simulink model "UPQC_original"  (R2020a)
settings: Solver=ode45  StartTime=0.0  StopTime=0.3  FixedStep=Ts  RelTol=1e-3  EnableMultiTasking=on
undefined symbols (not defined in the file or in its folder): DiscIntNeverNeededParam, Hydride, level, Metal, Nickel, sigbuilder_block
libraries: powerlib x73, powerlib_extras x9, simulink x7, powerlib_meascontrol x2, electricdrivelib x1, re_lib x1
(part 1 of 3)
settings Model: Creator=Dhamodharan  LastModifiedBy=User
settings DataIOCC: LimitDataPoints=on  SaveFormat=Array  ReturnWorkspaceOutputs=off
settings OptimizationCC: ExpressionDepthLimit=2147483647  InitFltsAndDblsToZero=on  LifeSpan=inf
settings DebuggingCC: SaveWithParameterizedLinksMsg=none  UnderspecifiedInitializationDetection=Classic  MergeDetectMultiDrivingBlocksExec=none  SignalResolutionControl=TryResolveAllWithWarning  SolverPrmCheckMsg=warning  MultiTaskDSMMsg=warning  MultiTaskCondExecSysMsg=none  FcnCallInpInsideContextMsg=warning  StateNameClashWarn=warning  SFUnexpectedBacktrackingDiag=warning  SFNoUnconditionalDefaultTransitionDiag=warning  SFExecutionAtInitializationDiag=none  ArithmeticOperatorsInVariantConditions=warning
settings HardwareCC: ProdBitPerPointer=32  ProdBitPerSizeT=32  ProdBitPerPtrDiffT=32  ProdLargestAtomicFloat=None  ProdIntDivRoundTo=Undefined  ProdEndianess=Unspecified  ProdWordSize=32  ProdHWDeviceType=32-bit Generic
settings ModelReferenceCC: PropagateSignalLabelsOutOfModel=off
settings SFSimCC: SimUseLocalCustomCode=off  CustomCodeUndefinedFunction=UseInterfaceOnly
settings RTWCC: RTWUseLocalCustomCode=off
settings CodeAppCC: StateflowObjectComments=on
settings GRTTargetCC: TargetFcnLib=ansi_tfl_tmw.mat  TargetLangStandard=C89/C90 (ANSI)  CombineOutputUpdateFcns=off  GRTInterface=on
settings ConfigComp: CovMetricSettings=dw  CovHtmlReporting=on  CovSaveCumulativeToWorkspaceVar=on  CovSaveSingleToWorkspaceVar=on  CovExternalEMLEnable=off
settings SimscapeCC: SimscapeNormalizeSystem=off

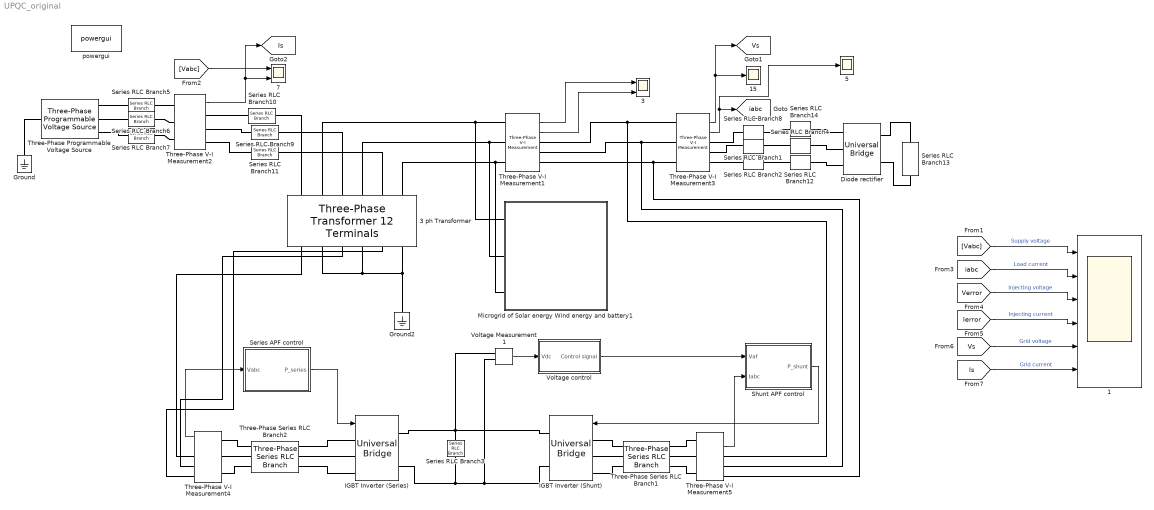
== system UPQC_original ==
  " IGBT Inverter (Series)" : powerlib/Power Electronics/Universal Bridge  Arms=3  SnubberResistance=5000  SnubberCapacitance=1e-6  Device=MOSFET / Diodes  Ron=1e-3  Lon=0  ForwardVoltages="[  0.1  0.1  ]"  ForwardVoltage=.8  GTOparameters=[ 1e-6 ,1e-6 ]  IGBTparameters=[ 1e-6 , 2e-6 ]  Measurements=Device currents  Measurements_2=None  converterType=Rectifier
  1 : Scope  NumInputPorts=6
  15 : Scope
  3 : Scope  NumInputPorts=2
  3 ph Transformer : powerlib/Elements/Three-Phase Transformer 12 Terminals  RatedPower=[ 10e6 50 ]  Winding1="[ 100 0.002  0.00005 ]"  Winding2=[ 100 0.002 0.00005]  RmXm=[ 200 200 ]
      settings: SourceProductBaseCode=PS
  5 : Scope
  7 : Scope  NumInputPorts=2
  Diode rectifier : powerlib/Power Electronics/Universal Bridge  Arms=3  SnubberResistance=1e5  SnubberCapacitance=inf  Device=Diodes  Ron=1e-3  Lon=0  ForwardVoltages="[  0  0  ]"  ForwardVoltage=0  GTOparameters=[ 10e-6 , 20e-6 ]  IGBTparameters=[ 1e-6 , 2e-6 ]  Measurements=None  Measurements_2=None  converterType=Rectifier
  Ground : powerlib/Elements/Ground  LConnTagsString=a
  Ground2 : powerlib/Elements/Ground  LConnTagsString=a
  IGBT Inverter (Shunt) : powerlib/Power Electronics/Universal Bridge  Arms=3  SnubberResistance=5000  SnubberCapacitance=1e-6  Device=MOSFET / Diodes  Ron=1e-3  Lon=0  ForwardVoltages="[  0.1  0.1  ]"  ForwardVoltage=.8  GTOparameters=[ 1e-6 ,1e-6 ]  IGBTparameters=[ 1e-6 , 2e-6 ]  Measurements=Device currents  Measurements_2=None  converterType=Rectifier
  Microgrid of Solar energy Wind energy and battery1 : Subsystem
  Series APF control : Subsystem
  Series RLC Branch{1..2,4,8,12,14} (6 alike) : powerlib/Elements/Series RLC Branch  LConnTagsString=__new0  RConnTagsString=__new0  BranchType=L  Resistance=1.0  Inductance=2e-3  SetiL0=off  InitialCurrent=0  Capacitance=1.0  Setx0=off  InitialVoltage=0  Measurements=None
  Series RLC Branch10 : powerlib/Elements/Series RLC Branch  LConnTagsString=__new0  RConnTagsString=__new0  BranchType=RL  Resistance=0.001  Inductance=1e-5  SetiL0=off  InitialCurrent=0  Capacitance=1.0  Setx0=off  InitialVoltage=0  Measurements=None
  Series RLC Branch11 : powerlib/Elements/Series RLC Branch  LConnTagsString=__new0  RConnTagsString=__new0  BranchType=RL  Resistance=0.001  Inductance=1e-5  SetiL0=off  InitialCurrent=0  Capacitance=1.0  Setx0=off  InitialVoltage=0  Measurements=None
  Series RLC Branch13 : powerlib/Elements/Series RLC Branch  LConnTagsString=__new0  RConnTagsString=__new0  BranchType=R  Resistance=40  Inductance=1e-4  SetiL0=off  InitialCurrent=0  Capacitance=1.0  Setx0=off  InitialVoltage=0  Measurements=None
  Series RLC Branch3 : powerlib/Elements/Series RLC Branch  LConnTagsString=__new0  RConnTagsString=__new0  BranchType=C  Resistance=1.0  Inductance=1.0  SetiL0=off  InitialCurrent=0  Capacitance=5  Setx0=on  InitialVoltage=800  Measurements=None
  Series RLC Branch5 : powerlib/Elements/Series RLC Branch  LConnTagsString=__new0  RConnTagsString=__new0  BranchType=R  Resistance=0.001  Inductance=1.0e-4  SetiL0=off  InitialCurrent=0  Capacitance=1.0  Setx0=off  InitialVoltage=0  Measurements=None
  Series RLC Branch6 : powerlib/Elements/Series RLC Branch  LConnTagsString=__new0  RConnTagsString=__new0  BranchType=R  Resistance=0.001  Inductance=1.0e-4  SetiL0=off  InitialCurrent=0  Capacitance=1.0  Setx0=off  InitialVoltage=0  Measurements=None
  Series RLC Branch7 : powerlib/Elements/Series RLC Branch  LConnTagsString=__new0  RConnTagsString=__new0  BranchType=R  Resistance=0.001  Inductance=1.0e-4  SetiL0=off  InitialCurrent=0  Capacitance=1.0  Setx0=off  InitialVoltage=0  Measurements=None
  Series RLC Branch9 : powerlib/Elements/Series RLC Branch  LConnTagsString=__new0  RConnTagsString=__new0  BranchType=RL  Resistance=0.001  Inductance=1e-5  SetiL0=off  InitialCurrent=0  Capacitance=1.0  Setx0=off  InitialVoltage=0  Measurements=None
  Shunt APF control : Subsystem
  Three-Phase Programmable Voltage Source : powerlib/Electrical Sources/Three-Phase Programmable Voltage Source  PositiveSequence="[230*sqrt(3)/sqrt(2)  0 50]"  VariationEntity=Amplitude  VariationType=Table of time-amplitude pairs  VariationTypeAlt=Step  VariationStep=0.5  VariationRate=10  VariationMagnitude=0.3  VariationFrequency=2  VariationTiming=[1 2]  VariationPhaseA=off  Amplitudes=[1 0.8 1.2 1]  TimeValues=[0 0.1 0.15 0.2]  HarmonicGeneration=on  HarmonicA=[5 0.2 -25 2]  HarmonicB=[7 0.2 35 1]  Timing="[0.25  0.4]"  BusType=swing  Pref=0  Qref=0  Qmin=-inf  Qmax=inf
  Three-Phase Series RLC Branch1 : powerlib/Elements/Three-Phase Series RLC Branch  LConnTagsString=A|B|C  RConnTagsString=A|B|C  BranchType=L  Resistance=0.  Inductance=3e-3  Capacitance=1e-6  Measurements=None
  Three-Phase Series RLC Branch2 : powerlib/Elements/Three-Phase Series RLC Branch  LConnTagsString=A|B|C  RConnTagsString=A|B|C  BranchType=L  Resistance=0.  Inductance=1e-3  Capacitance=1e-6  Measurements=None
  Three-Phase V-I Measurement1 : powerlib/Measurements/Three-Phase V-I Measurement  VoltageMeasurement=phase-to-ground  SetLabelV=off  LabelV=Vabc  Vpu=off  VpuLL=off  CurrentMeasurement=yes  SetLabelI=off  LabelI=Iabc  Ipu=off  Pbase=100e6  Vbase=500e3  OutputType=Complex  PhasorSimulation=off  PSBequivalent=0
  Three-Phase V-I Measurement2 : powerlib/Measurements/Three-Phase V-I Measurement  VoltageMeasurement=phase-to-ground  SetLabelV=on  LabelV=Vabc  Vpu=off  VpuLL=off  CurrentMeasurement=yes  SetLabelI=off  LabelI=Iabc  Ipu=off  Pbase=100e6  Vbase=500e3  OutputType=Complex  PhasorSimulation=off  PSBequivalent=0
  Three-Phase V-I Measurement3 : powerlib/Measurements/Three-Phase V-I Measurement  VoltageMeasurement=phase-to-ground  SetLabelV=off  LabelV=Vabc  Vpu=off  VpuLL=off  CurrentMeasurement=yes  SetLabelI=off  LabelI=Iabc  Ipu=off  Pbase=100e6  Vbase=500e3  OutputType=Complex  PhasorSimulation=off  PSBequivalent=0
  Three-Phase V-I Measurement4 : powerlib/Measurements/Three-Phase V-I Measurement  VoltageMeasurement=phase-to-ground  SetLabelV=off  LabelV=Vabc  Vpu=off  VpuLL=off  CurrentMeasurement=yes  SetLabelI=off  LabelI=Iabc  Ipu=off  Pbase=100e6  Vbase=500e3  OutputType=Complex  PhasorSimulation=off  PSBequivalent=0
  Three-Phase V-I Measurement5 : powerlib/Measurements/Three-Phase V-I Measurement  VoltageMeasurement=phase-to-phase  SetLabelV=off  LabelV=Vabc  Vpu=off  VpuLL=off  CurrentMeasurement=yes  SetLabelI=off  LabelI=Iabc  Ipu=off  Pbase=100e6  Vbase=500e3  OutputType=Complex  PhasorSimulation=off  PSBequivalent=0
  Voltage Measurement1 : powerlib/Measurements/Voltage Measurement  PhasorSimulation=off  OutputType=Complex  PSBequivalent=0
  Voltage control : Subsystem
  powergui : powerlib/powergui  SimulationMode=Discrete  SampleTime=8e-6  frequency=60  Iterations=50  frequencyindice=0  Pbase=100e6  ErrMax=1e-4  UnitsV=kV  UnitsW=MW  buscounter=0  FunctionMessages=off  echomessages=off  EnableUseOfTLC=off  CurrentSourceSwitches=off  DisableSnubberDevices=off  DisableRonSwitches=off  DisableVfSwitches=off  DisplayEquations=off  AutomaticDiscreteSolvers=off  SolverType=Tustin  Interpol=off  ExternalGateDelay=off  methode=off  Ts=0  x0status=blocks  SPID=off  SwTol=0  HookPort=off  NonlinearTolerance=1e-4  nMaxIteration=100  ContinueOnMaxIteration=off  RestoreLinks=warning  ResistiveCurrentMeasurement=off  Frange=[0:2:500]  Ylog=off  Xlog=on  ShowGrid=off  save=off  variable=ZData  structure=ScopeData2  ZoomFFT=off  StartTime=.1  cycles=1  DisplayStyle=1  fundamental=50  FreqAxis=off  MaxFrequency=1000  frequencyindicesteady=1  RmsSteady=1  display=off
  tag scope: Is=global, Vs=global, iabc=global
  wires:
  Three-Phase V-I Measurement3/2 -> [iabc], 5/1
  Three-Phase V-I Measurement2/1 -> [Is], 7/2
  [Vabc] -> 7/1
  Three-Phase V-I Measurement3/1 -> [Vs], 15/1
  Series APF control/1(P_series) -> " IGBT Inverter (Series)"/1
  Shunt APF control/1(P_shunt) -> IGBT Inverter (Shunt)/1
  [Vabc] -> 1/1  "Supply voltage"
  [iabc] -> 1/2  "Load current"
  [Verror] -> 1/3  "Injecting voltage"
  [Ierror] -> 1/4  "Injecting current"
  [Vs] -> 1/5  "Grid voltage"
  [Is] -> 1/6  "Grid current"
  Three-Phase V-I Measurement1/1 -> 3/1
  Three-Phase V-I Measurement1/2 -> 3/2
  Voltage Measurement1/1 -> Voltage control/1(Vdc)
  Voltage control/1("Control signal ") -> Shunt APF control/1(Vaf)
  Three-Phase V-I Measurement4/1 -> Series APF control/1(Vabc)
  Three-Phase V-I Measurement5/2 -> Shunt APF control/2(Iabc)
  connections:
  Series RLC Branch3/LConn1 -- " IGBT Inverter (Series)"/RConn1 -- Voltage Measurement1/LConn1 -- IGBT Inverter (Shunt)/RConn1
  Series RLC Branch3/RConn1 -- Voltage Measurement1/LConn2 -- IGBT Inverter (Shunt)/RConn2 -- " IGBT Inverter (Series)"/RConn2
  Series RLC Branch5/LConn1 -- Three-Phase Programmable Voltage Source/RConn1
  Series RLC Branch6/LConn1 -- Three-Phase Programmable Voltage Source/RConn2
  Series RLC Branch7/LConn1 -- Three-Phase Programmable Voltage Source/RConn3
  Series RLC Branch5/RConn1 -- Three-Phase V-I Measurement2/LConn1
  Series RLC Branch6/RConn1 -- Three-Phase V-I Measurement2/LConn2
  Series RLC Branch7/RConn1 -- Three-Phase V-I Measurement2/LConn3
  Three-Phase V-I Measurement3/RConn1 -- Series RLC Branch8/LConn1
  Three-Phase V-I Measurement3/RConn2 -- Series RLC Branch1/LConn1
  Series RLC Branch2/LConn1 -- Three-Phase V-I Measurement3/RConn3
  Three-Phase V-I Measurement2/RConn1 -- Series RLC Branch10/LConn1
  Three-Phase V-I Measurement2/RConn2 -- Series RLC Branch9/LConn1
  Three-Phase V-I Measurement2/RConn3 -- Series RLC Branch11/LConn1
  Series RLC Branch14/LConn1 -- Series RLC Branch8/RConn1
  Series RLC Branch4/LConn1 -- Series RLC Branch1/RConn1
  Series RLC Branch12/LConn1 -- Series RLC Branch2/RConn1
  Diode rectifier/RConn1 -- Series RLC Branch13/LConn1
  Diode rectifier/RConn2 -- Series RLC Branch13/RConn1
  Series RLC Branch12/RConn1 -- Diode rectifier/LConn3
  Series RLC Branch4/RConn1 -- Diode rectifier/LConn2
  Series RLC Branch14/RConn1 -- Diode rectifier/LConn1
  Ground/LConn1 -- Three-Phase Programmable Voltage Source/LConn1
  Three-Phase V-I Measurement1/RConn1 -- Three-Phase V-I Measurement5/RConn1 -- Three-Phase V-I Measurement3/LConn1
  Ground2/LConn1 -- 3 ph Transformer/LConn6 -- 3 ph Transformer/LConn4 -- 3 ph Transformer/LConn2
  " IGBT Inverter (Series)"/LConn1 -- Three-Phase Series RLC Branch2/LConn1
  " IGBT Inverter (Series)"/LConn2 -- Three-Phase Series RLC Branch2/LConn2
  " IGBT Inverter (Series)"/LConn3 -- Three-Phase Series RLC Branch2/LConn3
  3 ph Transformer/RConn1 -- Series RLC Branch10/RConn1
  3 ph Transformer/RConn3 -- Series RLC Branch9/RConn1
  Three-Phase V-I Measurement1/RConn2 -- Three-Phase V-I Measurement5/RConn2 -- Three-Phase V-I Measurement3/LConn2
  3 ph Transformer/RConn5 -- Series RLC Branch11/RConn1
  Three-Phase V-I Measurement1/RConn3 -- Three-Phase V-I Measurement5/RConn3 -- Three-Phase V-I Measurement3/LConn3
  IGBT Inverter (Shunt)/LConn1 -- Three-Phase Series RLC Branch1/LConn1
  Three-Phase Series RLC Branch1/LConn2 -- IGBT Inverter (Shunt)/LConn2
  IGBT Inverter (Shunt)/LConn3 -- Three-Phase Series RLC Branch1/LConn3
  Three-Phase V-I Measurement1/LConn1 -- Microgrid of Solar energy Wind energy and battery1/LConn1 -- 3 ph Transformer/RConn2
  Three-Phase V-I Measurement1/LConn2 -- Microgrid of Solar energy Wind energy and battery1/LConn2 -- 3 ph Transformer/RConn4
  Three-Phase V-I Measurement1/LConn3 -- Microgrid of Solar energy Wind energy and battery1/LConn3 -- 3 ph Transformer/RConn6
  Three-Phase V-I Measurement4/LConn3 -- Three-Phase Series RLC Branch2/RConn3
  Three-Phase V-I Measurement4/LConn2 -- Three-Phase Series RLC Branch2/RConn2
  Three-Phase Series RLC Branch2/RConn1 -- Three-Phase V-I Measurement4/LConn1
  Three-Phase Series RLC Branch1/RConn1 -- Three-Phase V-I Measurement5/LConn1
  Three-Phase V-I Measurement5/LConn2 -- Three-Phase Series RLC Branch1/RConn2
  Three-Phase V-I Measurement5/LConn3 -- Three-Phase Series RLC Branch1/RConn3
  Three-Phase V-I Measurement4/RConn1 -- 3 ph Transformer/LConn1
  Three-Phase V-I Measurement4/RConn2 -- 3 ph Transformer/LConn3
  Three-Phase V-I Measurement4/RConn3 -- 3 ph Transformer/LConn5

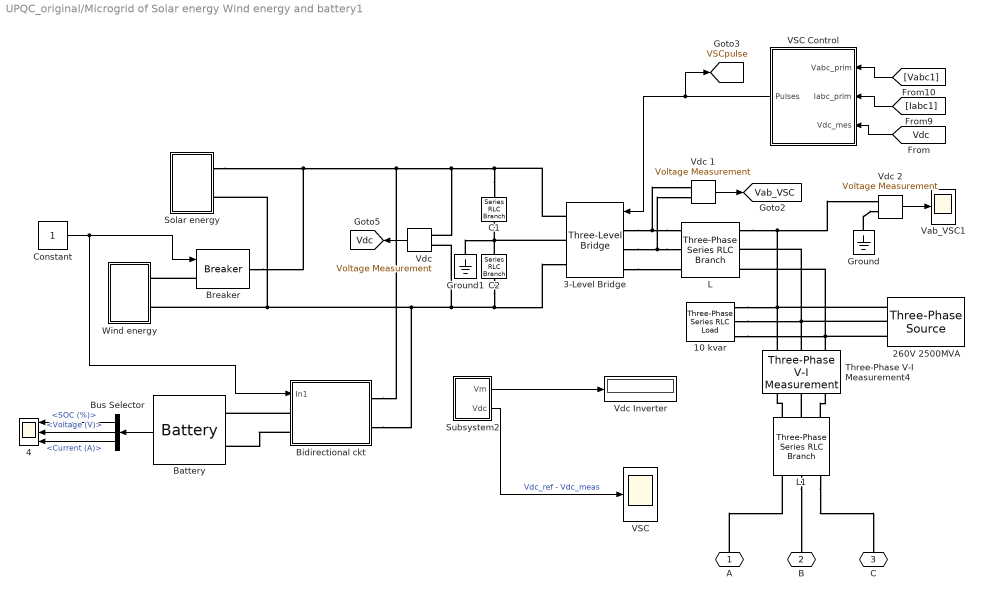
== system UPQC_original/Microgrid of Solar energy Wind energy and battery1 ==
  10 kvar : powerlib/Elements/Three-Phase Series RLC Load  LConnTagsString=A|B|C  Configuration=Y (grounded)  NominalVoltage=260  Vabc=[1e3 1e3 1e3]  Vabcp=[1e3 1e3 1e3]  NominalFrequency=50  UnbalancedPower=off  ActivePower=10e3/100  InductivePower=0  CapacitivePower=10e3  Pabc=[10e3 9e3 11e3]  QLabc=[100 90 110]  QCabc=[100 90 110]  Pabcp=[10e3 9e3 11e3]  QLabcp=[100 90 110]  QCabcp=[100 90 110]  Measurements=None  LoadType=constant Z
  260V 2500MVA : powerlib/Electrical Sources/Three-Phase Source  InternalConnection=Yg  VoltagePhases=off  Voltage=281  PhaseAngle=0  Voltage_phases=[25e3 25e3 25e3]/sqrt(3)  PhaseAngles_phases=[0 -120 +120]  Frequency=50  NonIdealSource=on  SpecifyImpedance=on  Resistance=0.8929  Inductance=16.58e-3  ShortCircuitLevel=2500e6  BaseVoltage=281  XRratio=7  BusType=swing  Pref=0  Qref=0  Prefabc=[10e3, 10e3, 10e3]  Qrefabc=[0, 0, 0]  Qmin=-inf  Qmax=inf
  3-Level Bridge : powerlib/Power Electronics/Three-Level Bridge  Arms=3  SnubberResistance=1e6  SbubberCapacitance=inf  Device=IGBT / Diodes  Ron=0.2e-3  ForwardVoltages="[  0  0 ]"  Measurements=None
      settings: SourceProductBaseCode=PS
  4 : Scope  NumInputPorts=3
  Battery : electricdrivelib/Extra Sources/Battery  BatType=Nickel-Metal-Hydride  ShowTempParam=off  ThermalPreset=no  ShowAgeParam=off  NomV=800  NomQ=10  SOC=20  Batt_Tr=30  PresetModel=on  MaxQ=10.7692  MinV=600  FullV=942.3729  Dis_rate=2  R=0.8  Normal_OP=9.6154  expZone="[867.7966             2]"  current=[1.5 3]  Units=Ampere-hour  Tci=20  NomT=20  T2=-30  MaxQ2=4.8  FullV2=7.1  Normal_OP2=5.655  expZone2="[6.58           1]"  Rca=0.6  ti=2000  Dp=0  Neq0=0  Tsim=1e6  Ta1=25  Qeol=5.4*0.9  Reol=0.013333*1.2  Char_age=[2.3478, 3]  Dis_age=[2.3478, 10]  N1=1500  N2=10500  N3=1000  N4=1400  Ta2=45  N5=950
  Bidirectional ckt : Subsystem
  Breaker : powerlib/Elements/Breaker  InitialState=0  SwitchingTimes="[ 1/60  5/60 ]"  External=on  BreakerResistance=0.01  SnubberResistance=1e6  SnubberCapacitance=inf  Measurements=None  MoreParameters=off  NoBreakLoop=off
  Bus Selector : BusSelector  OutputSignals=SOC (%),Voltage (V),Current (A)
  C1 : powerlib/Elements/Series RLC Branch  LConnTagsString=__new0  RConnTagsString=__new0  BranchType=C  Resistance=1.0  Inductance=1.0  SetiL0=off  InitialCurrent=0  Capacitance=12000e-06  Setx0=on  InitialVoltage=250  Measurements=None
  C2 : powerlib/Elements/Series RLC Branch  LConnTagsString=__new0  RConnTagsString=__new0  BranchType=C  Resistance=1.0  Inductance=1.0  SetiL0=off  InitialCurrent=0  Capacitance=12000e-06  Setx0=on  InitialVoltage=250  Measurements=None
  Constant : Constant
  Ground : powerlib/Elements/Ground  LConnTagsString=a
  Ground1 : powerlib/Elements/Ground  LConnTagsString=a
  L : powerlib/Elements/Three-Phase Series RLC Branch  LConnTagsString=A|B|C  RConnTagsString=A|B|C  BranchType=RL  Resistance=2e-6  Inductance=250e-5  Capacitance=inf  Measurements=None
  L1 : powerlib/Elements/Three-Phase Series RLC Branch  LConnTagsString=A|B|C  RConnTagsString=A|B|C  BranchType=R  Resistance=10  Inductance=250e-5  Capacitance=inf  Measurements=None
  Solar energy : Subsystem
  Subsystem2 : Subsystem
  Three-Phase V-I Measurement4 : powerlib/Measurements/Three-Phase V-I Measurement  VoltageMeasurement=phase-to-ground  SetLabelV=on  LabelV=Vabc4  Vpu=off  VpuLL=off  CurrentMeasurement=yes  SetLabelI=on  LabelI=Iabc4  Ipu=off  Pbase=100e6  Vbase=500e3  OutputType=Complex  PhasorSimulation=off  PSBequivalent=0
  VSC : Scope
  VSC Control : Subsystem  mask(VSC Main Controller){nom=[ 100e3  50 ], Vnom=[220 281], Vnom_dc=500, RLxfo=[0.002  0.06 ], RLchoke=[2e-3  250e-5 ], K_VDCreg=[7  800], K_Ireg=[0.3 20], Ts=1e-6}
      mask prompts: nom "Nominal power and frequency [ Pnom(VA)  Fnom(Hz) ]:"; Vnom "Nominal primary and secondary voltages (Vrms LL) [ Vnom_prim   Vnom_sec ]:"; Vnom_dc "Nominal DC bus voltage (V):"; RLxfo "Total transformer leakage impedance (pu/Pnom) [ Rxfo  Lxf ]"; RLchoke "Choke impedance [ R(ohm) L(H) ]"; K_VDCreg "VDC regultator gains [ Kp  Ki ]:"; K_Ireg "Current regulator gains [ Kp  Ki ]:"; Ts "Sample time"
      mask init:
      | Pnom=nom(1);
      | Fnom=nom(2);
      | Vnom_prim=Vnom(1);
      | Vnom_sec=Vnom(2);
      | Zbase=Vnom_sec^2/Pnom;
      | Rtot_pu=RLxfo(1) + RLchoke(1)/Zbase;
      | Ltot_pu=RLxfo(2) + RLchoke(2)/(Zbase/(2*pi*Fnom));
      | Kp_VDCreg=K_VDCreg(1);
      | Ki_VDCreg=K_VDCreg(2);
      | Kp_Ireg=K_Ireg(1);
      | Ki_Ireg=K_Ireg(2);
      | Vdc_ref=Vnom_dc;
  Vab_VSC1 : Scope
  "Vdc " : powerlib/Measurements/Voltage Measurement  Tag=PoWeRsYsTeMmEaSuReMeNt  PhasorSimulation=off  OutputType=Magnitude  PSBequivalent=0
  Vdc 1 : powerlib/Measurements/Voltage Measurement  Tag=PoWeRsYsTeMmEaSuReMeNt  PhasorSimulation=off  OutputType=Magnitude  PSBequivalent=0
  Vdc 2 : powerlib/Measurements/Voltage Measurement  Tag=PoWeRsYsTeMmEaSuReMeNt  PhasorSimulation=off  OutputType=Magnitude  PSBequivalent=0
  Vdc Inverter : Display
      settings: Format=bank  Decimation=2000
  Wind energy : Subsystem
  A : PMIOPort  Side=Left
  B : PMIOPort  Port=2  Side=Left
  "C " : PMIOPort  Port=3  Side=Left
  tag scope: VSCpulse=global, Vab_VSC=global, Vdc=global
  wires:
  Constant/1 -> Breaker/1, Bidirectional ckt/1(In1)
  Bus Selector/3 -> 4/3  "<Current (A)>"
  Bus Selector/2 -> 4/2  "<Voltage (V)>"
  Bus Selector/1 -> 4/1  "<SOC (%)>"
  Battery/1 -> Bus Selector/1
  VSC Control/1(Pulses) -> 3-Level Bridge/1, [VSCpulse]
  Vdc 2/1 -> Vab_VSC1/1
  Subsystem2/1(Vm) -> Vdc Inverter/1
  Subsystem2/2("Vdc ") -> VSC/1  "Vdc_ref - Vdc_meas"
  Vdc 1/1 -> [Vab_VSC]
  [Vdc] -> VSC Control/3(Vdc_mes)
  [Iabc1] -> VSC Control/2(Iabc_prim)
  [Vabc1] -> VSC Control/1(Vabc_prim)
  "Vdc "/1 -> [Vdc]
  connections:
  Bidirectional ckt/LConn2 -- Battery/LConn2
  Bidirectional ckt/LConn1 -- Battery/LConn1
  Breaker/LConn1 -- Wind energy/RConn1
  L1/RConn3 -- "C "/RConn1
  L1/RConn2 -- B/RConn1
  L1/LConn3 -- Three-Phase V-I Measurement4/RConn3
  L1/LConn2 -- Three-Phase V-I Measurement4/RConn2
  L1/LConn1 -- Three-Phase V-I Measurement4/RConn1
  A/RConn1 -- L1/RConn1
  Three-Phase V-I Measurement4/LConn1 -- L/RConn1 -- Vdc 2/LConn1 -- 260V 2500MVA/RConn1 -- 10 kvar/LConn1
  Three-Phase V-I Measurement4/LConn3 -- L/RConn3 -- 260V 2500MVA/RConn3 -- 10 kvar/LConn3
  Ground/LConn1 -- Vdc 2/LConn2
  Wind energy/RConn2 -- Solar energy/RConn2 -- Bidirectional ckt/RConn2 -- "Vdc "/LConn2 -- 3-Level Bridge/RConn3 -- C2/RConn1
  3-Level Bridge/LConn3 -- L/LConn3
  C1/RConn1 -- C2/LConn1 -- Ground1/LConn1 -- 3-Level Bridge/RConn2
  L/LConn2 -- 3-Level Bridge/LConn2 -- Vdc 1/LConn2
  L/LConn1 -- 3-Level Bridge/LConn1 -- Vdc 1/LConn1
  C1/LConn1 -- 3-Level Bridge/RConn1 -- Bidirectional ckt/RConn1 -- Solar energy/RConn1 -- Breaker/RConn1 -- "Vdc "/LConn1
  Three-Phase V-I Measurement4/LConn2 -- L/RConn2 -- 260V 2500MVA/RConn2 -- 10 kvar/LConn2

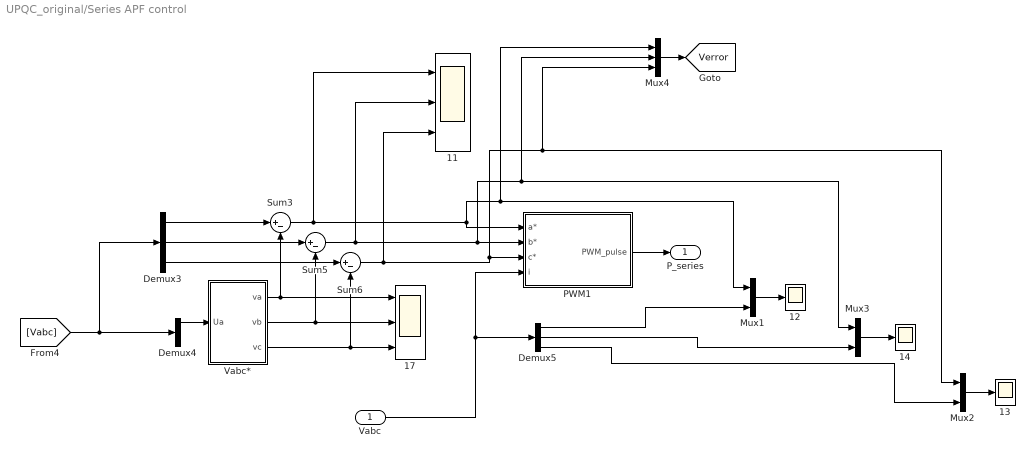
== system UPQC_original/Series APF control ==
  Vabc : Inport
  11 : Scope  NumInputPorts=3
  12 : Scope
  13 : Scope
  14 : Scope
  17 : Scope  NumInputPorts=3
  Demux3 : Demux  Outputs=3
      settings: DisplayOption=none
  Demux4 : Demux  Outputs=3
      settings: DisplayOption=none
  Demux5 : Demux  Outputs=3
      settings: DisplayOption=none
  Mux1 : Mux  Inputs=2
  Mux2 : Mux  Inputs=2
  Mux3 : Mux  Inputs=2
  Mux4 : Mux  Inputs=3
  PWM1 : Subsystem
  Sum3 : Sum  Inputs=|+-  SaturateOnIntegerOverflow=on
  Sum5 : Sum  Inputs=|+-  SaturateOnIntegerOverflow=on
  Sum6 : Sum  Inputs=|+-  SaturateOnIntegerOverflow=on
  Vabc* : Subsystem
  P_series : Outport  VectorParamsAs1DForOutWhenUnconnected=off
  tag scope: Verror=global
  wires:
  Demux3/1 -> Sum3/1
  Sum3/1 -> 11/1, PWM1/1(a*), Mux4/1, Mux1/1
  Vabc*/1(va) -> Sum3/2, 17/1
  Vabc*/2(vb) -> Sum5/2, 17/2
  Vabc*/3(vc) -> 17/3, Sum6/2
  Demux3/2 -> Sum5/1
  Demux3/3 -> Sum6/1
  Sum6/1 -> 11/3, PWM1/3(c*), Mux4/3, Mux2/1
  PWM1/1(PWM_pulse) -> P_series/1
  Demux4/1 -> Vabc*/1(Ua)
  [Vabc] -> Demux4/1, Demux3/1
  Vabc/1 -> PWM1/4(i), Demux5/1
  Sum5/1 -> 11/2, PWM1/2(b*), Mux4/2, Mux3/1
  Demux5/1 -> Mux1/2
  Mux1/1 -> 12/1
  Mux3/1 -> 14/1
  Demux5/2 -> Mux3/2
  Mux2/1 -> 13/1
  Demux5/3 -> Mux2/2
  Mux4/1 -> [Verror]

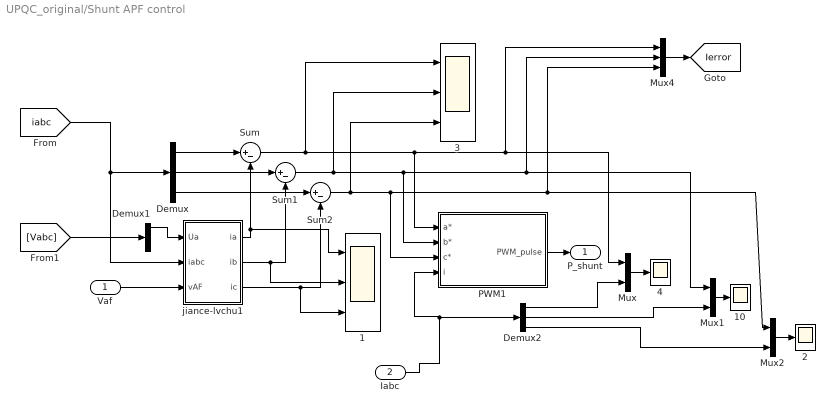
== system UPQC_original/Shunt APF control ==
  Vaf : Inport
  Iabc : Inport  Port=2
  1 : Scope  NumInputPorts=3
  10 : Scope
  2 : Scope
  3 : Scope  NumInputPorts=3
  4 : Scope
  Demux : Demux  Outputs=3
      settings: DisplayOption=none
  Demux1 : Demux  Outputs=3
      settings: DisplayOption=none
  Demux2 : Demux  Outputs=3
      settings: DisplayOption=none
  Mux : Mux  Inputs=2
  Mux1 : Mux  Inputs=2
  Mux2 : Mux  Inputs=2
  Mux4 : Mux  Inputs=3
  PWM1 : Subsystem
  Sum : Sum  Inputs=|+-  SaturateOnIntegerOverflow=on
  Sum1 : Sum  Inputs=|+-  SaturateOnIntegerOverflow=on
  Sum2 : Sum  Inputs=|+-  SaturateOnIntegerOverflow=on
  jiance-lvchu1 : Subsystem
  P_shunt : Outport  VectorParamsAs1DForOutWhenUnconnected=off
  tag scope: Ierror=global
  wires:
  Demux/1 -> Sum/1
  jiance-lvchu1/1(ia) -> Sum/2, 1/1
  jiance-lvchu1/2(ib) -> Sum1/2, 1/2
  jiance-lvchu1/3(ic) -> Sum2/2, 1/3
  Demux/2 -> Sum1/1
  Demux/3 -> Sum2/1
  [iabc] -> jiance-lvchu1/2(iabc), Demux/1
  [Vabc] -> Demux1/1
  PWM1/1(PWM_pulse) -> P_shunt/1
  Iabc/1 -> PWM1/4(i), Demux2/1
  Demux2/1 -> Mux/2
  Mux/1 -> 4/1
  Demux2/2 -> Mux1/2
  Mux1/1 -> 10/1
  Demux2/3 -> Mux2/2
  Mux2/1 -> 2/1
  Sum/1 -> 3/1, PWM1/1(a*), Mux4/1, Mux/1
  Sum2/1 -> 3/3, PWM1/3(c*), Mux4/3, Mux2/1
  Sum1/1 -> 3/2, PWM1/2(b*), Mux4/2, Mux1/1
  Mux4/1 -> [Ierror]
  Demux1/1 -> jiance-lvchu1/1(Ua)
  Vaf/1 -> jiance-lvchu1/3(vAF)

== system UPQC_original/Voltage control ==
  Vdc : Inport
  6 : Scope
  PID Controller : simulink/Continuous/PID Controller  Controller=PI  Form=Ideal  TimeDomain=Continuous-time  UseExternalTs=off  SampleTime=-1  IntegratorMethod=Forward Euler  FilterMethod=Forward Euler  ControllerParametersSource=internal  P=1  I=10  D=0  UseFilter=on  N=100  TunerSelectOption=Transfer Function Based (PID Tuner App)  InitialConditionSource=internal  InitialConditionForIntegrator=0  InitialConditionForFilter=0  DifferentiatorICPrevScaledInput=0  ExternalReset=none  TrackingMode=off  Kt=1  LimitOutput=off  UpperSaturationLimit=inf  LowerSaturationLimit=-inf  LinearizeAsGain=on  AntiWindupMode=none  Kb=1  POutMin=[]  POutMax=[]  IOutMin=[]  IOutMax=[]  DOutMin=[]  DOutMax=[]  NOutMin=[]  NOutMax=[]  SumOutMin=[]  SumOutMax=[]  SaturationOutMin=[]  SaturationOutMax=[]  PParamMin=[]  PParamMax=[]  IParamMin=[]  IParamMax=[]  DParamMin=[]  DParamMax=[]  NParamMin=[]  NParamMax=[]  KbParamMin=[]  KbParamMax=[]  KtParamMin=[]  KtParamMax=[]  KbOutMin=[]  KbOutMax=[]  KtOutMin=[]  KtOutMax=[]  IntegratorOutMin=[]  IntegratorOutMax=[]  FilterOutMin=[]  FilterOutMax=[]  SumI1OutMin=[]  SumI1OutMax=[]  SumI2OutMin=[]  SumI2OutMax=[]  SumI3OutMin=[]  SumI3OutMax=[]  SumI4OutMin=[]  SumI4OutMax=[]  SumDOutMin=[]  SumDOutMax=[]  DifferentiatorOutMin=[]  DifferentiatorOutMax=[]  FilterDiffOutCoefMin=[]  FilterDiffOutCoefMax=[]  ReciprocalOutMin=[]  ReciprocalOutMax=[]  SumDenOutMin=[]  SumDenOutMax=[]  SumNumOutMin=[]  SumNumOutMax=[]  DivideOutMin=[]  DivideOutMax=[]  UdiffTsProdOutMin=[]  UdiffTsProdOutMax=[]  NTsProdOutMin=[]  NTsProdOutMax=[]  UintegralTsProdOutMin=[]  UintegralTsProdOutMax=[]  UngainTsProdOutMin=[]  UngainTsProdOutMax=[]  IntegratorContinuousStateAttributes=''  IntegratorStateMustResolveToSignalObject=off  IntegratorRTWStateStorageClass=Auto  FilterContinuousStateAttributes=''  FilterStateMustResolveToSignalObject=off  FilterRTWStateStorageClass=Auto  ParallelPVariant=Passthrough  IdealPVariant=InternalParameters  IVariant=InternalParameters  DVariant=Disabled  IntegratorVariant=Continuous  SatVariant=Disabled  AWVariant=Passthrough  PCopyVariant=Disabled  TRVariant=Disabled  FdbkBlocksVariant=Forward  IdealPFdbkVariant=Disabled  SatFdbkVariant=Disabled  DerivativeFilterVariant=Disabled  NVariant=Disabled  NCopyVariant=Disabled_SignalSpec  FilterICVariant=Disabled  IntegratorICVariant=InternalICs  ExternalResetVariant=Disabled  TRSumVariant=Passthrough  SumFdbkVariant=Disabled  SumVariant=Sum_PI  TsampFilterVariant=InternalTs  TsampNgainVariant=Passthrough  TsampIntegralVariant=Passthrough
  Sum4 : Sum  Inputs=|+-  SaturateOnIntegerOverflow=on
  Vdc_ref : Constant  Value=800
  "Control signal " : Outport  VectorParamsAs1DForOutWhenUnconnected=off
  wires:
  Vdc_ref/1 -> Sum4/1
  Vdc/1 -> Sum4/2, 6/1
  PID Controller/1 -> "Control signal "/1
  Sum4/1 -> PID Controller/1  "in"

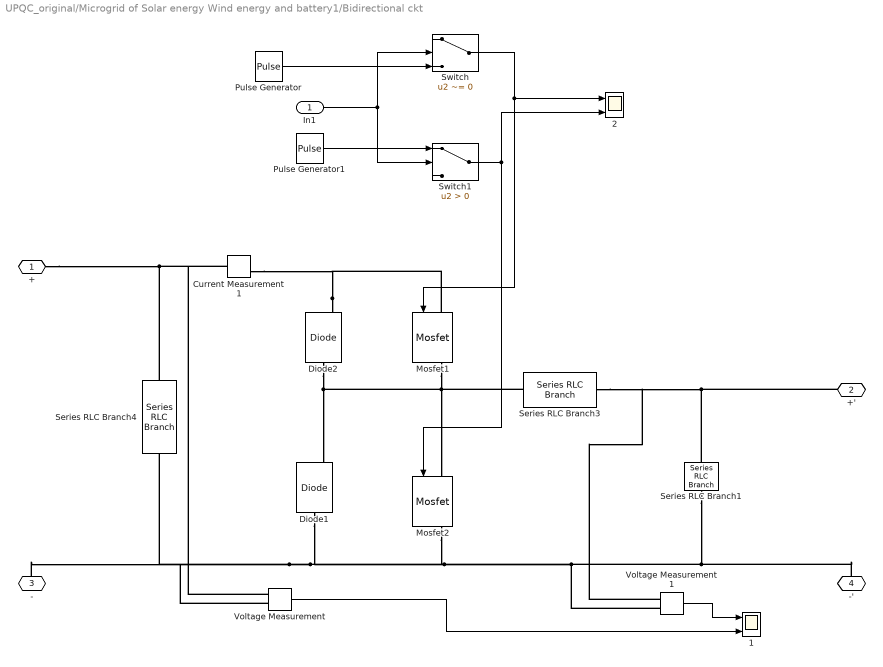
== system UPQC_original/Microgrid of Solar energy Wind energy and battery1/Bidirectional ckt ==
  In1 : Inport
  1 : Scope  NumInputPorts=2
  2 : Scope  NumInputPorts=2
  Current Measurement1 : powerlib/Measurements/Current Measurement  PhasorSimulation=off  OutputType=Complex  PSBequivalent=0
  Diode1 : powerlib/Power Electronics/Diode  Ron=0.001  Lon=0  Vf=0.1  IC=0  UseSnubber=off  Rs=500  Cs=250e-9  Measurements=on
  Diode2 : powerlib/Power Electronics/Diode  Ron=0.001  Lon=0  Vf=0.1  IC=0  UseSnubber=off  Rs=500  Cs=250e-9  Measurements=on
  Mosfet1 : powerlib/Power Electronics/Mosfet  Ron=0.1  Lon=0  Rd=0.01  Vfd=0  IC=0  Rs=1e5  Cs=inf  Measurements=on
  Mosfet2 : powerlib/Power Electronics/Mosfet  Ron=0.1  Lon=0  Rd=0.01  Vfd=0  IC=0  Rs=1e5  Cs=inf  Measurements=on
  Pulse Generator : DiscretePulseGenerator  PulseType=Time based  Period=1/20000  PulseWidth=55
  Pulse Generator1 : DiscretePulseGenerator  PulseType=Time based  Period=1/20000  PulseWidth=100-55
  Series RLC Branch1 : powerlib/Elements/Series RLC Branch  LConnTagsString=__new0  RConnTagsString=__new0  BranchType=C  Resistance=1  Inductance=1e-3  SetiL0=off  InitialCurrent=0  Capacitance=2.5e-4  Setx0=off  InitialVoltage=0  Measurements=None
  Series RLC Branch3 : powerlib/Elements/Series RLC Branch  LConnTagsString=__new0  RConnTagsString=__new0  BranchType=L  Resistance=1  Inductance=2.5e-4  SetiL0=off  InitialCurrent=0  Capacitance=1e-6  Setx0=off  InitialVoltage=0  Measurements=None
  Series RLC Branch4 : powerlib/Elements/Series RLC Branch  LConnTagsString=__new0  RConnTagsString=__new0  BranchType=C  Resistance=1  Inductance=1e-3  SetiL0=off  InitialCurrent=0  Capacitance=5e-4  Setx0=off  InitialVoltage=0  Measurements=None
  Switch : Switch  Criteria=u2 ~= 0
  Switch1 : Switch  Criteria=u2 > Threshold
  Voltage Measurement : powerlib/Measurements/Voltage Measurement  PhasorSimulation=off  OutputType=Complex  PSBequivalent=0
  Voltage Measurement1 : powerlib/Measurements/Voltage Measurement  PhasorSimulation=off  OutputType=Complex  PSBequivalent=0
  + : PMIOPort  Side=Left
  +' : PMIOPort  Port=2  Side=Right
  - : PMIOPort  Port=3  Side=Left
  -' : PMIOPort  Port=4  Side=Right
  wires:
  Voltage Measurement/1 -> 1/2
  Voltage Measurement1/1 -> 1/1
  Pulse Generator1/1 -> Switch1/1
  Pulse Generator/1 -> Switch/3
  In1/1 -> Switch/2, Switch1/2
  Switch/1 -> Mosfet1/1, 2/1
  Switch1/1 -> 2/2, Mosfet2/1
  connections:
  -'/RConn1 -- Series RLC Branch1/RConn1 -- Voltage Measurement1/LConn2 -- Diode1/LConn1 -- -/RConn1 -- Series RLC Branch4/RConn1 -- Voltage Measurement/LConn2 -- Mosfet2/RConn1
  +'/RConn1 -- Series RLC Branch1/LConn1 -- Voltage Measurement1/LConn1 -- Series RLC Branch3/RConn1
  +/RConn1 -- Current Measurement1/LConn1 -- Voltage Measurement/LConn1 -- Series RLC Branch4/LConn1
  Diode2/RConn1 -- Current Measurement1/RConn1 -- Mosfet1/LConn1
  Mosfet1/RConn1 -- Mosfet2/LConn1 -- Diode2/LConn1 -- Diode1/RConn1 -- Series RLC Branch3/LConn1
